simulink model "punto1"  (R2022a)
settings: Solver=VariableStepAuto  StartTime=0.0  StopTime=10.0  RelTol=1e-3
settings Model: Creator=juand  LastModifiedBy=juand

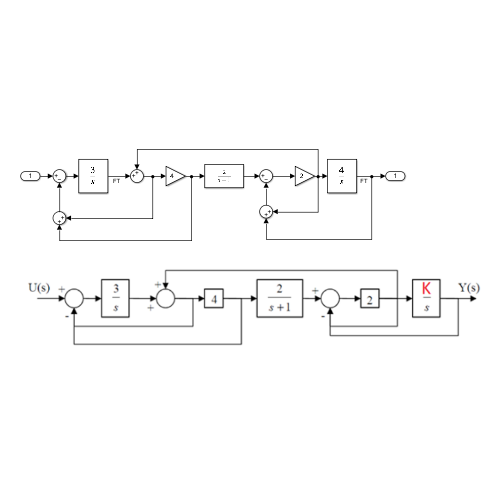
[thumbnail: Simulink's stored preview of the top-level diagram]
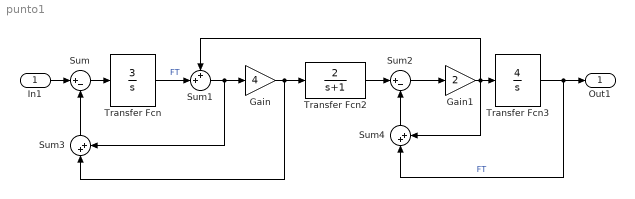
== system punto1 ==
  In1 : Inport
  Gain : Gain  Gain=4
  Gain1 : Gain  Gain=2
  Sum : Sum  Inputs=|+-
  Sum1 : Sum  Inputs=++|
  Sum2 : Sum  Inputs=|+-
  Sum3 : Sum  Inputs=|++
  Sum4 : Sum  Inputs=|++
  Transfer Fcn : TransferFcn  Numerator=[3]  Denominator=[1 0]
  Transfer Fcn2 : TransferFcn  Numerator=[2]  Denominator=[1 1]
  Transfer Fcn3 : TransferFcn  Numerator=[4]  Denominator=[1 0]
  Out1 : Outport
  wires:
  In1/1 -> Sum/1
  Sum/1 -> Transfer Fcn/1
  Transfer Fcn/1 -> Sum1/2  "FT"
  Transfer Fcn2/1 -> Sum2/1
  Transfer Fcn3/1 -> Sum4/1, Out1/1  "FT"
  Sum2/1 -> Gain1/1
  Sum1/1 -> Sum3/2, Gain/1
  Gain/1 -> Sum3/1, Transfer Fcn2/1
  Sum3/1 -> Sum/2
  Sum4/1 -> Sum2/2
  Gain1/1 -> Sum1/1, Sum4/2, Transfer Fcn3/1
